simulink model "model"  (R2024b)
settings: Solver=VariableStepAuto  StartTime=0.0  StopTime=inf  RelTol=1e-3
settings Model: Creator=deary  LastModifiedBy=deary

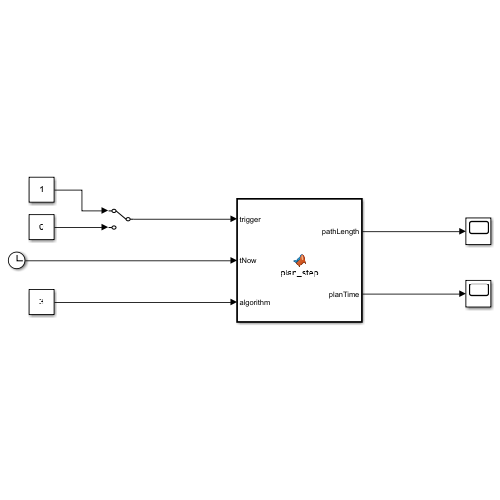
[thumbnail: Simulink's stored preview of the top-level diagram]
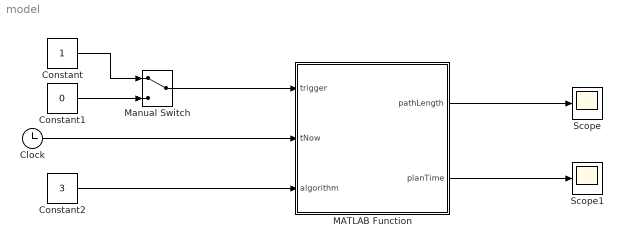
== system model ==
  Clock : Clock
  Constant : Constant
  Constant1 : Constant  Value=0
  Constant2 : Constant  Value=3
  MATLAB Function : MATLAB Function  TreatAsAtomicUnit=on
  Manual Switch : ManualSwitch
  Scope : Scope
  Scope1 : Scope
  wires:
  Clock/1 -> MATLAB Function/2(tNow)
  MATLAB Function/1(pathLength) -> Scope/1
  MATLAB Function/2(planTime) -> Scope1/1
  Manual Switch/1 -> MATLAB Function/1(trigger)
  Constant/1 -> Manual Switch/1
  Constant1/1 -> Manual Switch/2
  Constant2/1 -> MATLAB Function/3(algorithm)

== matlab function model/MATLAB Function ==
  data: trigger input; pathLength output; tNow input; algorithm input; planTime output
function [pathLength, planTime] = plan_step(trigger, tNow, algorithm)
coder.extrinsic('astar_3d_urban');
coder.extrinsic('rrt_star_3d_urban');
coder.extrinsic('prm_3d_urban');
coder.extrinsic('planner_visualizer');

% MATLAB Function block wrapper that:
%  - creates scenario once
%  - calls planners (A*, RRT*, PRM)
%  - computes path length + plan time
%  - updates a live 3-D viewer via an extrinsic helper

ReplanPeriod = 50;  

coder.extrinsic('planner_visualizer');

persistent scenario lastPlanTime lastTrig wps
if isempty(lastPlanTime)
    coder.varsize('wps',[10000,3],[true,false]);
    scenario = create_environment_3d();
    lastPlanTime = -inf;
    lastTrig = 0;
    wps = zeros(1,3);
end

pathLength = 0;
planTime   = 0;

trigRising = (trigger > 0.5) && (lastTrig <= 0.5);
lastTrig   = trigger;

% Replan if: rising edge OR period elapsed
if trigRising || (tNow - lastPlanTime) >= ReplanPeriod
    t0 = tic;
    switch round(algorithm)
        case 1
            wps = astar_3d_urban(scenario);
        case 2
            wps = rrt_star_3d_urban(scenario);
        otherwise
            wps = prm_3d_urban(scenario);
    end
    planTime = toc(t0);
    lastPlanTime = tNow;
end

% Compute length if we have a path
if ~isempty(wps) && size(wps,1) >= 2
    d = diff(wps);
    pathLength = sum(sqrt(sum(d.^2,2)));
else
    pathLength = 0;
end
planner_visualizer(scenario, wps, round(algorithm), tNow, pathLength, planTime);
